simulink model "Pt_All_4WD_TS801"  (Simulink 5.0)
settings: Solver=ode45  StartTime=0  StopTime=25  FixedStep=TSTEP  RelTol=1e-3
PreLoadFcn:
  | cd Extensions/Simulink/pt_all4wd
  | pt_parame_ft4wd
  | cd ../../..
values from neighbouring files (symbols this model uses):
  MENGINE_CARPET = [ ... (first row only)    [mengine_carpet.m]
undefined symbols (not defined in the file or in its folder): AV_ENG_IDLE, DOWNSHIFT_TRANS_TABLE_1, DOWNSHIFT_TRANS_TABLE_2, DOWNSHIFT_TRANS_TABLE_3, DOWNSHIFT_TRANS_TABLE_4, DOWNSHIFT_TRANS_TABLE_5, DOWNSHIFT_TRANS_TABLE_6, IENG, INV_CAP_TC_TABLE, ITC_INPUT_SHAFT, LOCKED_FD_DAMP, LOCKED_FD_K, LOCKED_FD_OPT, LOCKED_RD_DAMP, LOCKED_RD_K, LOCKED_RD_OPT, LOCKED_XC_DAMP, LOCKED_XC_K, LOCKED_XC_OPT, M_DIFF_FD_TABLE, M_DIFF_RD_TABLE, M_DIFF_XC_TABLE, R_EFF_F_FD, R_EFF_F_RD, R_EFF_F_XC, R_EFF_R_FD, R_EFF_R_RD, R_EFF_R_XC, R_EFF_TR_F, R_EFF_TR_F_REVERSE, R_EFF_TR_R, R_EFF_TR_R_REVERSE, R_GEAR_FD, R_GEAR_RD, R_GEAR_TR, R_GEAR_TR_REVERSE, R_GEAR_XC, R_REAR_XC, RM_TC_TABLE, UPSHIFT_TRANS_TABLE_1, UPSHIFT_TRANS_TABLE_2, UPSHIFT_TRANS_TABLE_3, UPSHIFT_TRANS_TABLE_4, UPSHIFT_TRANS_TABLE_5, UPSHIFT_TRANS_TABLE_6
libraries: Solver_SF x1
settings Model: LastModifiedBy=ywata  ExtModeTrigMode=oneshot  ExtModeArmWhenConnect=off  SaveTime=off  SaveOutput=off  LimitDataPoints=off  BooleanDataType=off

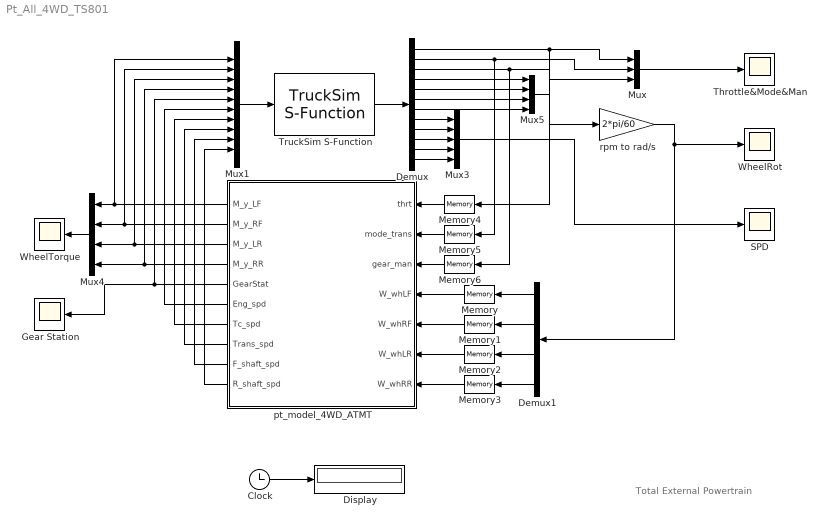
== system Pt_All_4WD_TS801 ==
  note: Total External Powertrain
  Clock : Clock
      settings: Decimation=10
  Demux : Demux  Outputs=12
  Demux1 : Demux  Orientation=left
  Display : Display
  Gear Station : Scope
      settings: YMin=0  YMax=6
  Memory{,1..6} (7 alike) : Memory  Orientation=left
  Mux : Mux  Inputs=3
  Mux1 : Mux  Inputs=10
  Mux3 : Mux  Inputs=5
  Mux4 : Mux  Orientation=left
  Mux5 : Mux
  SPD : Scope
      settings: TimeRange=25  YMin=-50  YMax=100
  Throttle&Mode&Man : Scope
      settings: YMin=0  YMax=7
  TruckSim S-Function : Solver_SF/TruckSim S-Function  Priority=1  AncestorBlock=Solver_SF/CarSim S-Function  VehicleCode=???
      settings: AttributesFormatString=Vehicle Code: %<VehicleCode>
  WheelRot : Scope
      settings: TimeRange=20  YMin=-10  YMax=50
  WheelTorque : Scope
      settings: YMin=0  YMax=2750
  pt_model_4WD_ATMT : Subsystem  Orientation=left
  rpm to rad/s : Gain  Gain=2*pi/60  SaturateOnIntegerOverflow=on
  wires:
  Mux1/1 -> TruckSim S-Function/1
  Mux/1 -> Throttle&Mode&Man/1
  Mux4/1 -> WheelTorque/1
  Demux/1 -> Mux/1, Memory4/1
  Demux/2 -> Mux/2, Memory5/1
  Demux/3 -> Mux/3, Memory6/1
  Demux1/1 -> Memory/1
  Demux1/2 -> Memory1/1
  Demux1/3 -> Memory2/1
  Demux1/4 -> Memory3/1
  Demux/5 -> Mux5/2
  Demux/6 -> Mux5/3
  Demux/4 -> Mux5/1
  Demux/7 -> Mux5/4
  Mux5/1 -> rpm to rad/s/1
  rpm to rad/s/1 -> Demux1/1, WheelRot/1
  Demux/8 -> Mux3/1
  Demux/9 -> Mux3/2
  Demux/10 -> Mux3/3
  Demux/11 -> Mux3/4
  Demux/12 -> Mux3/5
  Mux3/1 -> SPD/1
  pt_model_4WD_ATMT/1(M_y_LF) -> Mux1/1, Mux4/1
  pt_model_4WD_ATMT/2(M_y_RF) -> Mux1/2, Mux4/2
  pt_model_4WD_ATMT/3(M_y_LR) -> Mux4/3, Mux1/3
  pt_model_4WD_ATMT/4(M_y_RR) -> Mux4/4, Mux1/4
  pt_model_4WD_ATMT/5(GearStat) -> Gear Station/1, Mux1/5
  Clock/1 -> Display/1
  TruckSim S-Function/1 -> Demux/1
  Memory/1 -> pt_model_4WD_ATMT/4(W_whLF)
  Memory1/1 -> pt_model_4WD_ATMT/5(W_whRF)
  Memory2/1 -> pt_model_4WD_ATMT/6(W_whLR)
  Memory3/1 -> pt_model_4WD_ATMT/7(W_whRR)
  Memory4/1 -> pt_model_4WD_ATMT/1(thrt)
  Memory5/1 -> pt_model_4WD_ATMT/2(mode_trans)
  Memory6/1 -> pt_model_4WD_ATMT/3(gear_man)
  pt_model_4WD_ATMT/6(Eng_spd) -> Mux1/6
  pt_model_4WD_ATMT/7(Tc_spd) -> Mux1/7
  pt_model_4WD_ATMT/8(Trans_spd) -> Mux1/8
  pt_model_4WD_ATMT/9(F_shaft_spd) -> Mux1/9
  pt_model_4WD_ATMT/10(R_shaft_spd) -> Mux1/10

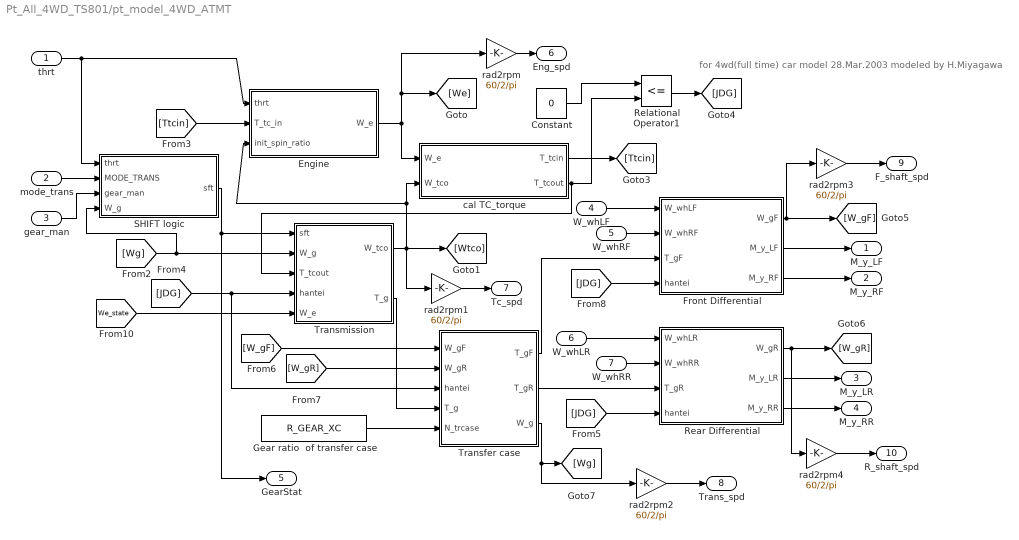
== system Pt_All_4WD_TS801/pt_model_4WD_ATMT ==
  note: for 4wd(full time) car model
      | 28.Mar.2003
      | modeled by H.Miyagawa
  thrt : Inport
  mode_trans : Inport  Port=2
  gear_man : Inport  Port=3
  W_whLF : Inport  Port=4
  W_whRF : Inport  Port=5
  W_whLR : Inport  Port=6
  W_whRR : Inport  Port=7
  Constant : Constant  Value=0
  Engine : Subsystem
  "Front Differential " : Subsystem
  Gear ratio  of transfer case : Constant  Value=R_GEAR_XC
  Rear Differential : Subsystem
  Relational Operator1 : RelationalOperator  Operator=<=  InputSameDT=on
  SHIFT logic : Subsystem
  Transfer case : Subsystem
  Transmission : Subsystem
  cal TC_torque : Subsystem
  rad2rpm{,1..4} (5 alike) : Gain  Gain=60/2/pi  SaturateOnIntegerOverflow=on
  M_y_LF : Outport
  M_y_RF : Outport  Port=2
  M_y_LR : Outport  Port=3
  M_y_RR : Outport  Port=4
  GearStat : Outport  Port=5
  Eng_spd : Outport  Port=6
  Tc_spd : Outport  Port=7
  Trans_spd : Outport  Port=8
  F_shaft_spd : Outport  Port=9
  R_shaft_spd : Outport  Port=10
  wires:
  SHIFT logic/1(sft) -> GearStat/1, Transmission/1(sft)
  [We_state] -> Transmission/5(W_e)
  Gear ratio  of transfer case/1 -> Transfer case/5(N_trcase)
  [W_gR] -> Transfer case/2(W_gR)
  [W_gF] -> Transfer case/1(W_gF)
  Transmission/2(T_g) -> Transfer case/4(T_g)
  [JDG] -> "Front Differential "/4(hantei)
  W_whLF/1 -> "Front Differential "/1(W_whLF)
  W_whRF/1 -> "Front Differential "/2(W_whRF)
  [JDG] -> Transfer case/3(hantei), Transmission/4(hantei)
  Transfer case/1(T_gF) -> "Front Differential "/3(T_gF)
  "Front Differential "/3(M_y_RF) -> M_y_RF/1
  "Front Differential "/2(M_y_LF) -> M_y_LF/1
  cal TC_torque/1(T_tcin) -> [Ttcin]
  cal TC_torque/2(T_tcout) -> Transmission/3(T_tcout), Relational Operator1/2
  [Wg] -> SHIFT logic/4(W_g), Transmission/2(W_g)
  Relational Operator1/1 -> [JDG]
  [Ttcin] -> Engine/2(T_tc_in)
  Transmission/1(W_tco) -> cal TC_torque/2(W_tco), Engine/3(init_spin_ratio), [Wtco], rad2rpm1/1
  Engine/1(W_e) -> cal TC_torque/1(W_e), [We], rad2rpm/1
  mode_trans/1 -> SHIFT logic/2(MODE_TRANS)
  gear_man/1 -> SHIFT logic/3(gear_man)
  thrt/1 -> SHIFT logic/1(thrt), Engine/1(thrt)
  Transfer case/3(W_g) -> [Wg], rad2rpm2/1
  "Front Differential "/1(W_gF) -> [W_gF], rad2rpm3/1
  Transfer case/2(T_gR) -> Rear Differential/3(T_gR)
  Rear Differential/3(M_y_RR) -> M_y_RR/1
  Rear Differential/2(M_y_LR) -> M_y_LR/1
  W_whRR/1 -> Rear Differential/2(W_whRR)
  W_whLR/1 -> Rear Differential/1(W_whLR)
  [JDG] -> Rear Differential/4(hantei)
  Rear Differential/1(W_gR) -> [W_gR], rad2rpm4/1
  rad2rpm/1 -> Eng_spd/1
  rad2rpm1/1 -> Tc_spd/1
  rad2rpm2/1 -> Trans_spd/1
  rad2rpm3/1 -> F_shaft_spd/1
  rad2rpm4/1 -> R_shaft_spd/1
  Constant/1 -> Relational Operator1/1

== system Pt_All_4WD_TS801/pt_model_4WD_ATMT/Engine ==
  thrt : Inport
  T_tc_in : Inport  Port=2
  init_spin_ratio : Inport  Port=3
  Spin inertia of engine crankshaft (kg-m2) : Constant  Value=IENG
  Spin inertia of input shaft of torque converter (kg-m2) : Constant  Value=ITC_INPUT_SHAFT
  cal Engine_torque : Subsystem
  cal We : Subsystem
  W_e : Outport
  wires:
  cal Engine_torque/1(T_e) -> cal We/1(T_e)
  cal We/1(We) -> W_e/1, cal Engine_torque/1(We)
  thrt/1 -> cal Engine_torque/2(thrt)
  init_spin_ratio/1 -> cal We/5(init spin ratio)
  T_tc_in/1 -> cal We/2(T_tc_in)
  Spin inertia of input shaft of torque converter (kg-m2)/1 -> cal We/4(I_tc_in)
  Spin inertia of engine crankshaft (kg-m2)/1 -> cal We/3(I_e)

== system Pt_All_4WD_TS801/pt_model_4WD_ATMT/Front Differential  ==
  W_whLF : Inport
  W_whRF : Inport  Port=2
  T_gF : Inport  Port=3
  hantei : Inport  Port=4
  Differeneial Gear : Subsystem
  Gear ratio of front differential : Constant  Value=R_GEAR_FD
  haibun : Subsystem
  W_gF : Outport
  M_y_LF : Outport  Port=2
  M_y_RF : Outport  Port=3
  wires:
  haibun/2(M_y_RF) -> M_y_RF/1
  haibun/1(M_y_LF) -> M_y_LF/1
  W_whRF/1 -> Differeneial Gear/2(W_whRF), haibun/2(W_whRF)
  W_whLF/1 -> Differeneial Gear/1(W_whLF), haibun/1(W_whLF)
  Gear ratio of front differential/1 -> haibun/5(N_diff_F), Differeneial Gear/3(N_diff_F)
  Differeneial Gear/1(W_g) -> W_gF/1
  T_gF/1 -> haibun/4(T_gF)
  hantei/1 -> haibun/3(hantei)

== system Pt_All_4WD_TS801/pt_model_4WD_ATMT/Rear Differential ==
  W_whLR : Inport
  W_whRR : Inport  Port=2
  T_gR : Inport  Port=3
  hantei : Inport  Port=4
  Differeneial Gear : Subsystem
  Gear ratio of rear differential : Constant  Value=R_GEAR_RD
  haibun : Subsystem
  W_gR : Outport
  M_y_LR : Outport  Port=2
  M_y_RR : Outport  Port=3
  wires:
  hantei/1 -> haibun/3(hantei)
  T_gR/1 -> haibun/4(T_gR)
  Differeneial Gear/1(W_g) -> W_gR/1
  Gear ratio of rear differential/1 -> Differeneial Gear/3(N_diff_R), haibun/5(N_diff_R)
  W_whLR/1 -> haibun/1(W_whLR), Differeneial Gear/1(W_whLR)
  W_whRR/1 -> haibun/2(W_whRR), Differeneial Gear/2(W_whRR)
  haibun/1(M_y_LR) -> M_y_LR/1
  haibun/2(M_y_RR) -> M_y_RR/1

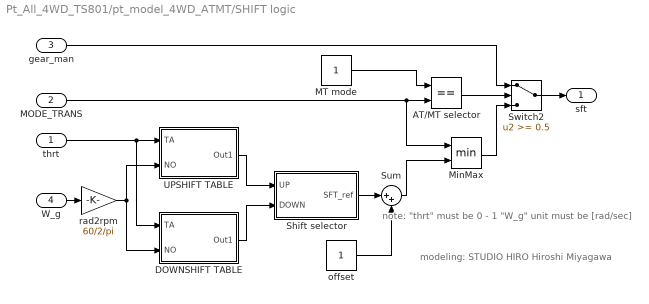
== system Pt_All_4WD_TS801/pt_model_4WD_ATMT/SHIFT logic ==
  note: note:
      | "thrt" must be 0 - 1
      | "W_g" unit must be [rad/sec]
  note: modeling:
      | STUDIO HIRO
      | Hiroshi Miyagawa
  thrt : Inport
  MODE_TRANS : Inport  Port=2
  gear_man : Inport  Port=3
  W_g : Inport  Port=4
  AT/MT selector : RelationalOperator  Operator===  InputSameDT=on
  DOWNSHIFT TABLE : Subsystem
  MT mode : Constant
  MinMax : MinMax  Inputs=2
  Shift selector : Subsystem
  Sum : Sum  Inputs=|++  SaturateOnIntegerOverflow=on  InputSameDT=on
  Switch2 : Switch  Threshold=0.5  SaturateOnIntegerOverflow=on  InputSameDT=on
  UPSHIFT TABLE : Subsystem
  offset : Constant
  rad2rpm : Gain  Gain=60/2/pi  SaturateOnIntegerOverflow=on
  sft : Outport
  wires:
  MinMax/1 -> Switch2/3
  AT/MT selector/1 -> Switch2/2
  gear_man/1 -> Switch2/1
  MODE_TRANS/1 -> MinMax/1, AT/MT selector/2
  MT mode/1 -> AT/MT selector/1
  thrt/1 -> DOWNSHIFT TABLE/1(TA), UPSHIFT TABLE/1(TA)
  Sum/1 -> MinMax/2
  W_g/1 -> rad2rpm/1
  DOWNSHIFT TABLE/1(Out1) -> Shift selector/2(DOWN)
  UPSHIFT TABLE/1(Out1) -> Shift selector/1(UP)
  rad2rpm/1 -> DOWNSHIFT TABLE/2(NO), UPSHIFT TABLE/2(NO)
  Shift selector/1(SFT_ref) -> Sum/1
  offset/1 -> Sum/2
  Switch2/1 -> sft/1

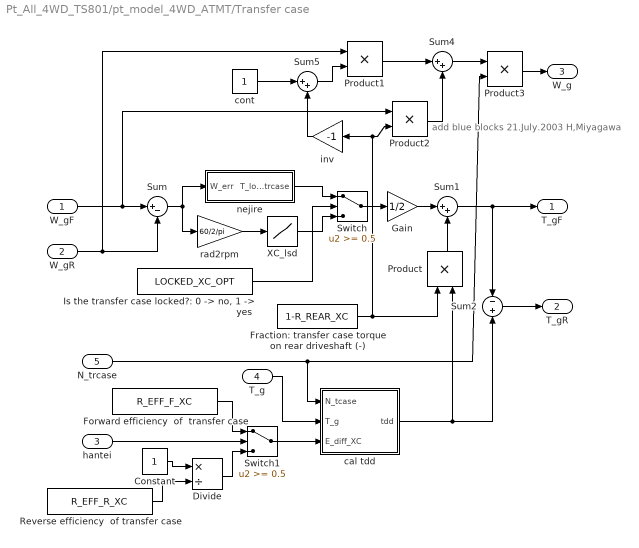
== system Pt_All_4WD_TS801/pt_model_4WD_ATMT/Transfer case ==
  note: add blue blocks
      | 21.July.2003
      | H,Miyagawa
  W_gF : Inport
  W_gR : Inport  Port=2
  hantei : Inport  Port=3
  T_g : Inport  Port=4
  N_trcase : Inport  Port=5
  Constant : Constant
  Divide : Product  Inputs=*/  InputSameDT=on
  Forward efficiency  of  transfer case : Constant  Value=R_EFF_F_XC
  Fraction: transfer case torque on rear driveshaft (-) : Constant  Value=1-R_REAR_XC
  Gain : Gain  Gain=1/2  SaturateOnIntegerOverflow=on
  "Is the transfer case locked?: 0 -> no, 1 -> yes" : Constant  Value=LOCKED_XC_OPT
  Product : Product  Orientation=up  SaturateOnIntegerOverflow=on  InputSameDT=on
  Product1 : Product  SaturateOnIntegerOverflow=on  InputSameDT=on
  Product2 : Product  SaturateOnIntegerOverflow=on  InputSameDT=on
  Product3 : Product  SaturateOnIntegerOverflow=on  InputSameDT=on
  Reverse efficiency  of transfer case : Constant  Value=R_EFF_R_XC
  Sum : Sum  Inputs=|+-  SaturateOnIntegerOverflow=on  InputSameDT=on
  Sum1 : Sum  Inputs=|++  SaturateOnIntegerOverflow=on  InputSameDT=on
  Sum2 : Sum  Inputs=-|+  SaturateOnIntegerOverflow=on  InputSameDT=on
  Sum4 : Sum  Inputs=|++  SaturateOnIntegerOverflow=on  InputSameDT=on
  Sum5 : Sum  Inputs=|++  SaturateOnIntegerOverflow=on  InputSameDT=on
  Switch : Switch  Threshold=0.5  SaturateOnIntegerOverflow=on  InputSameDT=on
  Switch1 : Switch  Threshold=0.5  SaturateOnIntegerOverflow=on  InputSameDT=on
  XC_lsd : Lookup  InputValues=M_DIFF_XC_TABLE(:,1)  OutputValues=M_DIFF_XC_TABLE(:,2)  SaturateOnIntegerOverflow=on
  cal tdd : Subsystem
  cont : Constant
  inv : Gain  Orientation=left  Gain=-1  SaturateOnIntegerOverflow=on
  nejire : Subsystem
  rad2rpm : Gain  Gain=60/2/pi  SaturateOnIntegerOverflow=on
  T_gF : Outport
  T_gR : Outport  Port=2
  W_g : Outport  Port=3
  wires:
  Sum1/1 -> Sum2/1, T_gF/1
  Sum2/1 -> T_gR/1
  cal tdd/1(tdd) -> Product/2, Sum2/2
  Switch1/1 -> cal tdd/3(E_diff_XC)
  Forward efficiency  of  transfer case/1 -> Switch1/1
  hantei/1 -> Switch1/2
  T_g/1 -> cal tdd/2(T_g)
  Product/1 -> Sum1/2
  Gain/1 -> Sum1/1
  Switch/1 -> Gain/1
  XC_lsd/1 -> Switch/3
  "Is the transfer case locked?: 0 -> no, 1 -> yes"/1 -> Switch/2
  Sum/1 -> rad2rpm/1, nejire/1(W_err)
  rad2rpm/1 -> XC_lsd/1
  nejire/1(T_lock_trcase) -> Switch/1
  Fraction: transfer case torque on rear driveshaft (-)/1 -> Product/1, Product2/2, inv/1
  Product2/1 -> Sum4/2
  Product1/1 -> Sum4/1
  Sum4/1 -> Product3/1
  Product3/1 -> W_g/1
  N_trcase/1 -> cal tdd/1(N_tcase), Product3/2
  Sum5/1 -> Product1/2
  cont/1 -> Sum5/1
  inv/1 -> Sum5/2
  W_gF/1 -> Sum/1, Product2/1
  W_gR/1 -> Sum/2, Product1/1
  Constant/1 -> Divide/1
  Reverse efficiency  of transfer case/1 -> Divide/2
  Divide/1 -> Switch1/3

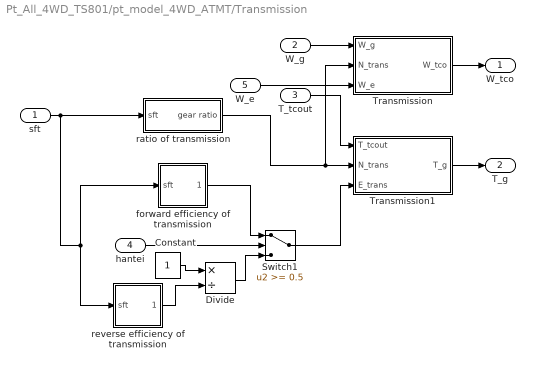
== system Pt_All_4WD_TS801/pt_model_4WD_ATMT/Transmission ==
  sft : Inport
  W_g : Inport  Port=2
  T_tcout : Inport  Port=3
  hantei : Inport  Port=4
  W_e : Inport  Port=5
  Constant : Constant
  Divide : Product  Inputs=*/  InputSameDT=on
  Switch1 : Switch  Threshold=0.5  SaturateOnIntegerOverflow=on  InputSameDT=on
  Transmission : Subsystem
  Transmission1 : Subsystem
  forward efficiency of transmission : Subsystem  mask(forward efficiency of transmission){data=R_EFF_TR_F, data_rev=R_EFF_TR_F_REVERSE}
      mask prompts: data "gear"; data_rev "Reverse-gear"
  ratio of transmission : Subsystem  mask(forward efficiency of transmission){data=R_GEAR_TR, data_rev=R_GEAR_TR_REVERSE}
      mask prompts: data "gear ratio"; data_rev "Reverse-gear ratio"
      mask help:
      | input:
      |  sft is must be 0 - 7
      | output:
      |  transmission gear ratio
      |  when Nutral(0), it is zero
      | 1st parameta:
      |  must be vector
      | 2nd parameter:
      |  should be negative
  reverse efficiency of transmission : Subsystem  mask(reverse efficiency of transmission){data=R_EFF_TR_R, data_rev=R_EFF_TR_R_REVERSE}
      mask prompts: data "gear"; data_rev "Reverse-gear"
  W_tco : Outport
  T_g : Outport  Port=2
  wires:
  W_e/1 -> Transmission/3(W_e)
  forward efficiency of transmission/1(Out1) -> Switch1/1
  hantei/1 -> Switch1/2
  ratio of transmission/1(gear ratio) -> Transmission1/2(N_trans), Transmission/2(N_trans)
  W_g/1 -> Transmission/1(W_g)
  Transmission1/1(T_g) -> T_g/1
  T_tcout/1 -> Transmission1/1(T_tcout)
  Switch1/1 -> Transmission1/3(E_trans)
  sft/1 -> ratio of transmission/1(sft), reverse efficiency of transmission/1(sft), forward efficiency of transmission/1(sft)
  Transmission/1(W_tco) -> W_tco/1
  Constant/1 -> Divide/1
  reverse efficiency of transmission/1(Out1) -> Divide/2
  Divide/1 -> Switch1/3

== system Pt_All_4WD_TS801/pt_model_4WD_ATMT/cal TC_torque ==
  note: Torque Convertor input & output torque calculation
  W_e : Inport
  W_tco : Inport  Port=2
  Math Function : Math  Operator=square
  Product : Product  SaturateOnIntegerOverflow=on  InputSameDT=on
  Product1 : Product  SaturateOnIntegerOverflow=on  InputSameDT=on
  Product2 : Product  SaturateOnIntegerOverflow=on  InputSameDT=on
  Sign : Signum
  cal speed_ratio : Subsystem
  f_tki : Lookup  InputValues=INV_CAP_TC_TABLE(:,1)  OutputValues=INV_CAP_TC_TABLE(:,2)  SaturateOnIntegerOverflow=on
  f_tr : Lookup  InputValues=RM_TC_TABLE(:,1)  OutputValues=RM_TC_TABLE(:,2)  SaturateOnIntegerOverflow=on
  rad2rpm : Gain  Gain=60/2/pi  SaturateOnIntegerOverflow=on
  T_tcin : Outport
  T_tcout : Outport  Port=2
  wires:
  Product/1 -> Math Function/1
  f_tki/1 -> Product/1, Sign/1
  Math Function/1 -> Product1/2
  Sign/1 -> Product1/1
  W_e/1 -> cal speed_ratio/2(W_e), rad2rpm/1
  cal speed_ratio/1(S_tc) -> f_tki/1, f_tr/1
  f_tr/1 -> Product2/2
  Product1/1 -> Product2/1, T_tcin/1
  W_tco/1 -> cal speed_ratio/1(W_tco)
  Product2/1 -> T_tcout/1
  rad2rpm/1 -> Product/2

== system Pt_All_4WD_TS801/pt_model_4WD_ATMT/Engine/cal Engine_torque ==
  We : Inport
  thrt : Inport  Port=2
  f_et : Lookup2D  RowIndex=MENGINE_CARPET(2:18,1)  ColumnIndex=MENGINE_CARPET(1,2:12)  OutputValues=MENGINE_CARPET(2:18,2:12)  SaturateOnIntegerOverflow=on  InputSameDT=on
  rad2rpm : Gain  Gain=60/2/pi  SaturateOnIntegerOverflow=on
  T_e : Outport
  wires:
  rad2rpm/1 -> f_et/1
  We/1 -> rad2rpm/1
  f_et/1 -> T_e/1
  thrt/1 -> f_et/2

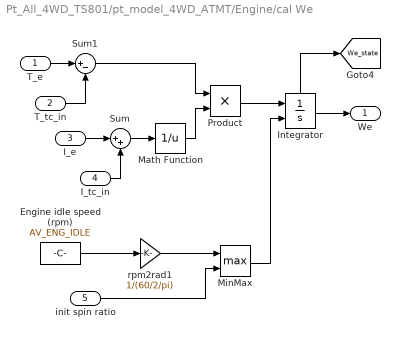
== system Pt_All_4WD_TS801/pt_model_4WD_ATMT/Engine/cal We ==
  T_e : Inport
  T_tc_in : Inport  Port=2
  I_e : Inport  Port=3
  I_tc_in : Inport  Port=4
  init spin ratio : Inport  Port=5
  Engine idle speed (rpm) : Constant  Value=AV_ENG_IDLE
  Integrator : Integrator  InitialConditionSource=external  InitialCondition=AV_ENG_IDLE*2*pi/60  ShowStatePort=on
  Math Function : Math  Operator=reciprocal
  MinMax : MinMax  Function=max  Inputs=2
  Product : Product  SaturateOnIntegerOverflow=on  InputSameDT=on
  Sum : Sum  Inputs=|++  SaturateOnIntegerOverflow=on  InputSameDT=on
  Sum1 : Sum  Inputs=|+-  SaturateOnIntegerOverflow=on  InputSameDT=on
  rpm2rad1 : Gain  Gain=1/(60/2/pi)  SaturateOnIntegerOverflow=on
  We : Outport
  tag scope: We_state=global
  wires:
  Integrator/State -> [We_state]
  MinMax/1 -> Integrator/2
  rpm2rad1/1 -> MinMax/1
  Engine idle speed (rpm)/1 -> rpm2rad1/1
  init spin ratio/1 -> MinMax/2
  Integrator/1 -> We/1
  Product/1 -> Integrator/1
  I_tc_in/1 -> Sum/2
  I_e/1 -> Sum/1
  T_tc_in/1 -> Sum1/2
  Sum/1 -> Math Function/1
  T_e/1 -> Sum1/1
  Sum1/1 -> Product/1
  Math Function/1 -> Product/2

== system Pt_All_4WD_TS801/pt_model_4WD_ATMT/Front Differential /Differeneial Gear ==
  W_whLF : Inport
  W_whRF : Inport  Port=2
  N_diff_F : Inport  Port=3
  Gain1 : Gain  Gain=1/2  SaturateOnIntegerOverflow=on
  Product : Product  SaturateOnIntegerOverflow=on  InputSameDT=on
  Sum : Sum  Inputs=|++  SaturateOnIntegerOverflow=on  InputSameDT=on
  W_g : Outport
  wires:
  Product/1 -> W_g/1
  Gain1/1 -> Product/1
  W_whRF/1 -> Sum/2
  W_whLF/1 -> Sum/1
  N_diff_F/1 -> Product/2
  Sum/1 -> Gain1/1

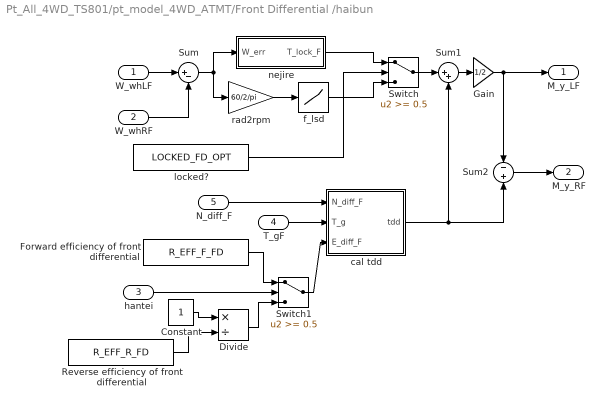
== system Pt_All_4WD_TS801/pt_model_4WD_ATMT/Front Differential /haibun ==
  W_whLF : Inport
  W_whRF : Inport  Port=2
  hantei : Inport  Port=3
  T_gF : Inport  Port=4
  N_diff_F : Inport  Port=5
  Constant : Constant
  Divide : Product  Inputs=*/  InputSameDT=on
  Forward efficiency of front differential : Constant  Value=R_EFF_F_FD
  Gain : Gain  Gain=1/2  SaturateOnIntegerOverflow=on
  Reverse efficiency of front differential : Constant  Value=R_EFF_R_FD
  Sum : Sum  Inputs=|+-  SaturateOnIntegerOverflow=on  InputSameDT=on
  Sum1 : Sum  Inputs=|++  SaturateOnIntegerOverflow=on  InputSameDT=on
  Sum2 : Sum  Inputs=-|+  SaturateOnIntegerOverflow=on  InputSameDT=on
  Switch : Switch  Threshold=0.5  SaturateOnIntegerOverflow=on  InputSameDT=on
  Switch1 : Switch  Threshold=0.5  SaturateOnIntegerOverflow=on  InputSameDT=on
  cal tdd : Subsystem
  f_lsd : Lookup  InputValues=M_DIFF_FD_TABLE(:,1)  OutputValues=M_DIFF_FD_TABLE(:,2)  SaturateOnIntegerOverflow=on
  locked? : Constant  Value=LOCKED_FD_OPT
  nejire : Subsystem
  rad2rpm : Gain  Gain=60/2/pi  SaturateOnIntegerOverflow=on
  M_y_LF : Outport
  M_y_RF : Outport  Port=2
  wires:
  T_gF/1 -> cal tdd/2(T_g)
  hantei/1 -> Switch1/2
  Forward efficiency of front differential/1 -> Switch1/1
  Switch1/1 -> cal tdd/3(E_diff_F)
  W_whLF/1 -> Sum/1
  W_whRF/1 -> Sum/2
  cal tdd/1(tdd) -> Sum1/2, Sum2/2
  Sum2/1 -> M_y_RF/1
  N_diff_F/1 -> cal tdd/1(N_diff_F)
  nejire/1(T_lock_F) -> Switch/1
  Switch/1 -> Sum1/1
  rad2rpm/1 -> f_lsd/1
  Sum1/1 -> Gain/1
  Gain/1 -> M_y_LF/1, Sum2/1
  Sum/1 -> nejire/1(W_err), rad2rpm/1
  locked?/1 -> Switch/2
  f_lsd/1 -> Switch/3
  Constant/1 -> Divide/1
  Reverse efficiency of front differential/1 -> Divide/2
  Divide/1 -> Switch1/3

== system Pt_All_4WD_TS801/pt_model_4WD_ATMT/Rear Differential/Differeneial Gear ==
  W_whLR : Inport
  W_whRR : Inport  Port=2
  N_diff_R : Inport  Port=3
  Gain1 : Gain  Gain=1/2  SaturateOnIntegerOverflow=on
  Product : Product  SaturateOnIntegerOverflow=on  InputSameDT=on
  Sum : Sum  Inputs=|++  SaturateOnIntegerOverflow=on  InputSameDT=on
  W_g : Outport
  wires:
  Sum/1 -> Gain1/1
  N_diff_R/1 -> Product/2
  W_whLR/1 -> Sum/1
  W_whRR/1 -> Sum/2
  Gain1/1 -> Product/1
  Product/1 -> W_g/1

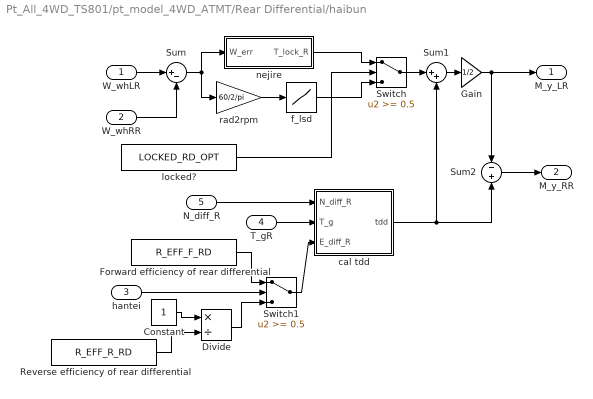
== system Pt_All_4WD_TS801/pt_model_4WD_ATMT/Rear Differential/haibun ==
  W_whLR : Inport
  W_whRR : Inport  Port=2
  hantei : Inport  Port=3
  T_gR : Inport  Port=4
  N_diff_R : Inport  Port=5
  Constant : Constant
  Divide : Product  Inputs=*/  InputSameDT=on
  Forward efficiency of rear differential : Constant  Value=R_EFF_F_RD
  Gain : Gain  Gain=1/2  SaturateOnIntegerOverflow=on
  Reverse efficiency of rear differential : Constant  Value=R_EFF_R_RD
  Sum : Sum  Inputs=|+-  SaturateOnIntegerOverflow=on  InputSameDT=on
  Sum1 : Sum  Inputs=|++  SaturateOnIntegerOverflow=on  InputSameDT=on
  Sum2 : Sum  Inputs=-|+  SaturateOnIntegerOverflow=on  InputSameDT=on
  Switch : Switch  Threshold=0.5  SaturateOnIntegerOverflow=on  InputSameDT=on
  Switch1 : Switch  Threshold=0.5  SaturateOnIntegerOverflow=on  InputSameDT=on
  cal tdd : Subsystem
  f_lsd : Lookup  InputValues=M_DIFF_RD_TABLE(:,1)  OutputValues=M_DIFF_RD_TABLE(:,2)  SaturateOnIntegerOverflow=on
  locked? : Constant  Value=LOCKED_RD_OPT
  nejire : Subsystem
  rad2rpm : Gain  Gain=60/2/pi  SaturateOnIntegerOverflow=on
  M_y_LR : Outport
  M_y_RR : Outport  Port=2
  wires:
  f_lsd/1 -> Switch/3
  locked?/1 -> Switch/2
  Sum/1 -> rad2rpm/1, nejire/1(W_err)
  Gain/1 -> Sum2/1, M_y_LR/1
  Sum1/1 -> Gain/1
  rad2rpm/1 -> f_lsd/1
  Switch/1 -> Sum1/1
  nejire/1(T_lock_R) -> Switch/1
  N_diff_R/1 -> cal tdd/1(N_diff_R)
  Sum2/1 -> M_y_RR/1
  cal tdd/1(tdd) -> Sum2/2, Sum1/2
  W_whRR/1 -> Sum/2
  W_whLR/1 -> Sum/1
  Switch1/1 -> cal tdd/3(E_diff_R)
  Forward efficiency of rear differential/1 -> Switch1/1
  hantei/1 -> Switch1/2
  T_gR/1 -> cal tdd/2(T_g)
  Constant/1 -> Divide/1
  Reverse efficiency of rear differential/1 -> Divide/2
  Divide/1 -> Switch1/3

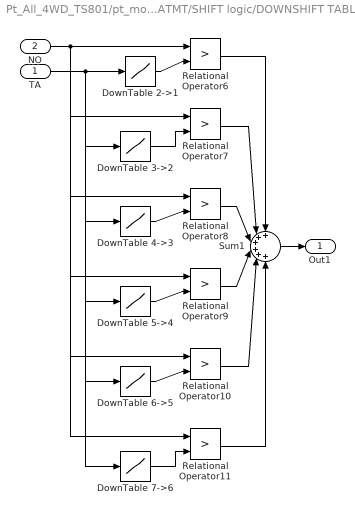
== system Pt_All_4WD_TS801/pt_model_4WD_ATMT/SHIFT logic/DOWNSHIFT TABLE ==
  TA : Inport
  NO : Inport  Port=2
  DownTable 2->1 : Lookup  InputValues=DOWNSHIFT_TRANS_TABLE_1(:,1)  OutputValues=DOWNSHIFT_TRANS_TABLE_1(:,2)  SaturateOnIntegerOverflow=on
  DownTable 3->2 : Lookup  InputValues=DOWNSHIFT_TRANS_TABLE_2(:,1)  OutputValues=DOWNSHIFT_TRANS_TABLE_2(:,2)  SaturateOnIntegerOverflow=on
  DownTable 4->3 : Lookup  InputValues=DOWNSHIFT_TRANS_TABLE_3(:,1)  OutputValues=DOWNSHIFT_TRANS_TABLE_3(:,2)  SaturateOnIntegerOverflow=on
  DownTable 5->4 : Lookup  InputValues=DOWNSHIFT_TRANS_TABLE_4(:,1)  OutputValues=DOWNSHIFT_TRANS_TABLE_4(:,2)  SaturateOnIntegerOverflow=on
  DownTable 6->5 : Lookup  InputValues=DOWNSHIFT_TRANS_TABLE_5(:,1)  OutputValues=DOWNSHIFT_TRANS_TABLE_5(:,2)  SaturateOnIntegerOverflow=on
  DownTable 7->6 : Lookup  InputValues=DOWNSHIFT_TRANS_TABLE_6(:,1)  OutputValues=DOWNSHIFT_TRANS_TABLE_6(:,2)  SaturateOnIntegerOverflow=on
  Relational Operator{6..11} (6 alike) : RelationalOperator  Operator=>  InputSameDT=on
  Sum1 : Sum  Inputs=6  SaturateOnIntegerOverflow=on  InputSameDT=on
  Out1 : Outport
  wires:
  Sum1/1 -> Out1/1
  NO/1 -> Relational Operator11/1, Relational Operator10/1, Relational Operator9/1, Relational Operator8/1, Relational Operator7/1, Relational Operator6/1
  TA/1 -> DownTable 7->6/1, DownTable 6->5/1, DownTable 5->4/1, DownTable 4->3/1, DownTable 3->2/1, DownTable 2->1/1
  DownTable 7->6/1 -> Relational Operator11/2
  DownTable 6->5/1 -> Relational Operator10/2
  DownTable 5->4/1 -> Relational Operator9/2
  DownTable 3->2/1 -> Relational Operator7/2
  DownTable 2->1/1 -> Relational Operator6/2
  Relational Operator11/1 -> Sum1/6
  Relational Operator10/1 -> Sum1/5
  Relational Operator9/1 -> Sum1/4
  Relational Operator8/1 -> Sum1/3
  Relational Operator7/1 -> Sum1/2
  Relational Operator6/1 -> Sum1/1
  DownTable 4->3/1 -> Relational Operator8/2

== system Pt_All_4WD_TS801/pt_model_4WD_ATMT/SHIFT logic/Shift selector ==
  UP : Inport
  DOWN : Inport  Port=2
  Logical Operator2 : Logic  Operator=OR
  Memory : Memory  Orientation=left
  Relational Operator2 : RelationalOperator  Operator=>  InputSameDT=on
  Relational Operator3 : RelationalOperator  Operator=>  InputSameDT=on
  Switch : Switch  Threshold=0.5  SaturateOnIntegerOverflow=on  InputSameDT=on
  Switch1 : Switch  Threshold=0.5  SaturateOnIntegerOverflow=on  InputSameDT=on
  SFT_ref : Outport
  wires:
  DOWN/1 -> Switch1/3, Relational Operator3/2
  UP/1 -> Switch1/1, Relational Operator2/1
  Relational Operator3/1 -> Logical Operator2/2
  Relational Operator2/1 -> Logical Operator2/1, Switch1/2
  Logical Operator2/1 -> Switch/2
  [SFT] -> Relational Operator3/1, Relational Operator2/2
  Memory/1 -> [SFT], Switch/3
  Switch1/1 -> Switch/1
  Switch/1 -> SFT_ref/1, Memory/1

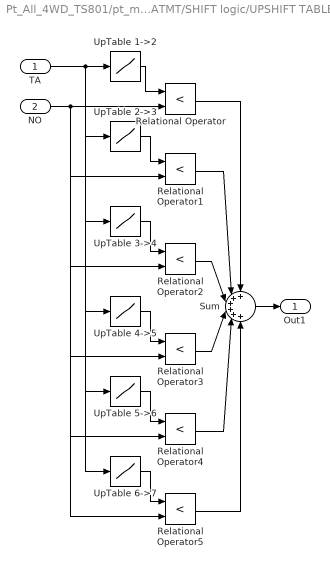
== system Pt_All_4WD_TS801/pt_model_4WD_ATMT/SHIFT logic/UPSHIFT TABLE ==
  TA : Inport
  NO : Inport  Port=2
  Relational Operator{,1..5} (6 alike) : RelationalOperator  Operator=<  InputSameDT=on
  Sum : Sum  Inputs=6  SaturateOnIntegerOverflow=on  InputSameDT=on
  UpTable 1->2 : Lookup  InputValues=UPSHIFT_TRANS_TABLE_1(:,1)  OutputValues=UPSHIFT_TRANS_TABLE_1(:,2)  SaturateOnIntegerOverflow=on
  UpTable 2->3 : Lookup  InputValues=UPSHIFT_TRANS_TABLE_2(:,1)  OutputValues=UPSHIFT_TRANS_TABLE_2(:,2)  SaturateOnIntegerOverflow=on
  UpTable 3->4 : Lookup  InputValues=UPSHIFT_TRANS_TABLE_3(:,1)  OutputValues=UPSHIFT_TRANS_TABLE_3(:,2)  SaturateOnIntegerOverflow=on
  UpTable 4->5 : Lookup  InputValues=UPSHIFT_TRANS_TABLE_4(:,1)  OutputValues=UPSHIFT_TRANS_TABLE_4(:,2)  SaturateOnIntegerOverflow=on
  UpTable 5->6 : Lookup  InputValues=UPSHIFT_TRANS_TABLE_5(:,1)  OutputValues=UPSHIFT_TRANS_TABLE_5(:,2)  SaturateOnIntegerOverflow=on
  UpTable 6->7 : Lookup  InputValues=UPSHIFT_TRANS_TABLE_6(:,1)  OutputValues=UPSHIFT_TRANS_TABLE_6(:,2)  SaturateOnIntegerOverflow=on
  Out1 : Outport
  wires:
  Sum/1 -> Out1/1
  NO/1 -> Relational Operator5/2, Relational Operator4/2, Relational Operator3/2, Relational Operator2/2, Relational Operator1/2, Relational Operator/2
  TA/1 -> UpTable 6->7/1, UpTable 5->6/1, UpTable 4->5/1, UpTable 3->4/1, UpTable 2->3/1, UpTable 1->2/1
  Relational Operator5/1 -> Sum/6
  Relational Operator4/1 -> Sum/5
  Relational Operator3/1 -> Sum/4
  Relational Operator2/1 -> Sum/3
  Relational Operator1/1 -> Sum/2
  Relational Operator/1 -> Sum/1
  UpTable 6->7/1 -> Relational Operator5/1
  UpTable 5->6/1 -> Relational Operator4/1
  UpTable 4->5/1 -> Relational Operator3/1
  UpTable 3->4/1 -> Relational Operator2/1
  UpTable 2->3/1 -> Relational Operator1/1
  UpTable 1->2/1 -> Relational Operator/1

== system Pt_All_4WD_TS801/pt_model_4WD_ATMT/Transfer case/cal tdd ==
  N_tcase : Inport
  T_g : Inport  Port=2
  E_diff_XC : Inport  Port=3
  Gain : Gain  SaturateOnIntegerOverflow=on
  Product : Product  Inputs=3  SaturateOnIntegerOverflow=on  InputSameDT=on
  tdd : Outport
  wires:
  T_g/1 -> Product/1
  N_tcase/1 -> Product/2
  E_diff_XC/1 -> Product/3
  Product/1 -> Gain/1
  Gain/1 -> tdd/1

== system Pt_All_4WD_TS801/pt_model_4WD_ATMT/Transfer case/nejire ==
  W_err : Inport
  Gain : Gain  Gain=-1  SaturateOnIntegerOverflow=on
  Integrator1 : Integrator
  Product : Product  SaturateOnIntegerOverflow=on  InputSameDT=on
  Product1 : Product  SaturateOnIntegerOverflow=on  InputSameDT=on
  Sum1 : Sum  Inputs=|++  SaturateOnIntegerOverflow=on  InputSameDT=on
  Torsional damping constant for locking the transfer case (N-m-s/deg) : Constant  Value=LOCKED_XC_DAMP
  Torsional spring constant for locking the transfer case (N-m/deg) : Constant  Value=LOCKED_XC_K
  rad2deg : Gain  Gain=360/2/pi  SaturateOnIntegerOverflow=on
  T_lock_trcase : Outport
  wires:
  Torsional spring constant for locking the transfer case (N-m/deg)/1 -> Product1/2
  Integrator1/1 -> Product1/1
  Torsional damping constant for locking the transfer case (N-m-s/deg)/1 -> Product/2
  Product/1 -> Sum1/1
  Product1/1 -> Sum1/2
  Sum1/1 -> Gain/1
  Gain/1 -> T_lock_trcase/1
  W_err/1 -> rad2deg/1
  rad2deg/1 -> Product/1, Integrator1/1

== system Pt_All_4WD_TS801/pt_model_4WD_ATMT/Transmission/Transmission ==
  W_g : Inport
  N_trans : Inport  Port=2
  W_e : Inport  Port=3
  Constant : Constant  Value=0
  Constant1 : Constant  Value=0
  MinMax : MinMax  Function=max  Inputs=2
  Product : Product  SaturateOnIntegerOverflow=on  InputSameDT=on
  Relational Operator : RelationalOperator  Operator===  InputSameDT=on
  Switch : Switch  Threshold=0.5  SaturateOnIntegerOverflow=on  InputSameDT=on
  W_tco : Outport
  wires:
  MinMax/1 -> Switch/3
  Product/1 -> MinMax/1
  Constant1/1 -> MinMax/2
  Switch/1 -> W_tco/1
  N_trans/1 -> Relational Operator/2, Product/1
  Constant/1 -> Relational Operator/1
  W_e/1 -> Switch/1
  Relational Operator/1 -> Switch/2
  W_g/1 -> Product/2

== system Pt_All_4WD_TS801/pt_model_4WD_ATMT/Transmission/Transmission1 ==
  T_tcout : Inport
  N_trans : Inport  Port=2
  E_trans : Inport  Port=3
  Product : Product  Inputs=3  SaturateOnIntegerOverflow=on  InputSameDT=on
  T_g : Outport
  wires:
  N_trans/1 -> Product/2
  T_tcout/1 -> Product/1
  E_trans/1 -> Product/3
  Product/1 -> T_g/1

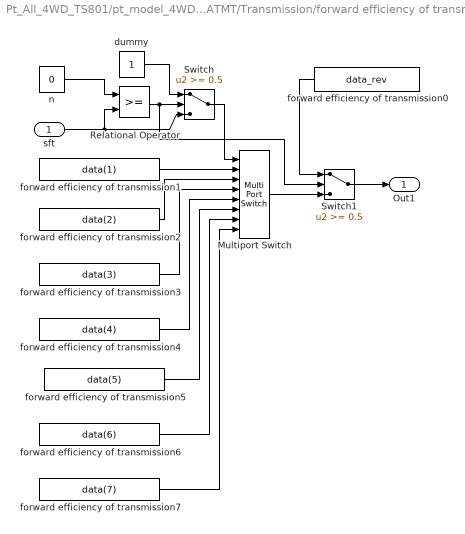
== system Pt_All_4WD_TS801/pt_model_4WD_ATMT/Transmission/forward efficiency of transmission ==
  sft : Inport
  Multiport Switch : MultiPortSwitch  Inputs=7  SaturateOnIntegerOverflow=on  InputSameDT=on
  Relational Operator : RelationalOperator  InputSameDT=on
  Switch : Switch  Threshold=0.5  SaturateOnIntegerOverflow=on  InputSameDT=on
  Switch1 : Switch  Threshold=0.5  SaturateOnIntegerOverflow=on  InputSameDT=on
  dummy : Constant
  forward efficiency of transmission0 : Constant  Orientation=left  Value=data_rev
  forward efficiency of transmission1 : Constant  Value=data(1)
  forward efficiency of transmission2 : Constant  Value=data(2)
  forward efficiency of transmission3 : Constant  Value=data(3)
  forward efficiency of transmission4 : Constant  Value=data(4)
  forward efficiency of transmission5 : Constant  Value=data(5)
  forward efficiency of transmission6 : Constant  Value=data(6)
  forward efficiency of transmission7 : Constant  Value=data(7)
  n : Constant  Value=0
  Out1 : Outport
  wires:
  dummy/1 -> Switch/1
  forward efficiency of transmission0/1 -> Switch1/1
  Relational Operator/1 -> Switch1/2, Switch/2
  n/1 -> Relational Operator/1
  sft/1 -> Switch/3, Relational Operator/2
  Multiport Switch/1 -> Switch1/3
  Switch1/1 -> Out1/1
  forward efficiency of transmission7/1 -> Multiport Switch/8
  forward efficiency of transmission6/1 -> Multiport Switch/7
  forward efficiency of transmission5/1 -> Multiport Switch/6
  forward efficiency of transmission4/1 -> Multiport Switch/5
  forward efficiency of transmission3/1 -> Multiport Switch/4
  forward efficiency of transmission2/1 -> Multiport Switch/3
  Switch/1 -> Multiport Switch/1
  forward efficiency of transmission1/1 -> Multiport Switch/2

== system Pt_All_4WD_TS801/pt_model_4WD_ATMT/Transmission/ratio of transmission ==
  sft : Inport
  1st-gear ratio of transmission : Constant  Value=data(1)
  2nd-gear ratio of transmission2 : Constant  Value=data(2)
  3rd-gear ratio of transmission3 : Constant  Value=data(3)
  4th-gear ratio of transmission4 : Constant  Value=data(4)
  5th-gear ratio of transmission5 : Constant  Value=data(5)
  6th-gear ratio of transmission6 : Constant  Value=data(6)
  7th-gear ratio of transmission7 : Constant  Value=data(7)
  Multiport Switch : MultiPortSwitch  Inputs=9  SaturateOnIntegerOverflow=on  InputSameDT=on
  N : Constant  Value=0
  Reverse-gear ratio of transmission1 : Constant  Value=data_rev
  Sum : Sum  Inputs=2  SaturateOnIntegerOverflow=on  InputSameDT=on
  off set : Constant  Value=2
  gear ratio : Outport
  wires:
  N/1 -> Multiport Switch/3
  Sum/1 -> Multiport Switch/1
  Reverse-gear ratio of transmission1/1 -> Multiport Switch/2
  7th-gear ratio of transmission7/1 -> Multiport Switch/10
  6th-gear ratio of transmission6/1 -> Multiport Switch/9
  5th-gear ratio of transmission5/1 -> Multiport Switch/8
  4th-gear ratio of transmission4/1 -> Multiport Switch/7
  3rd-gear ratio of transmission3/1 -> Multiport Switch/6
  2nd-gear ratio of transmission2/1 -> Multiport Switch/5
  1st-gear ratio of transmission/1 -> Multiport Switch/4
  Multiport Switch/1 -> gear ratio/1
  off set/1 -> Sum/1
  sft/1 -> Sum/2

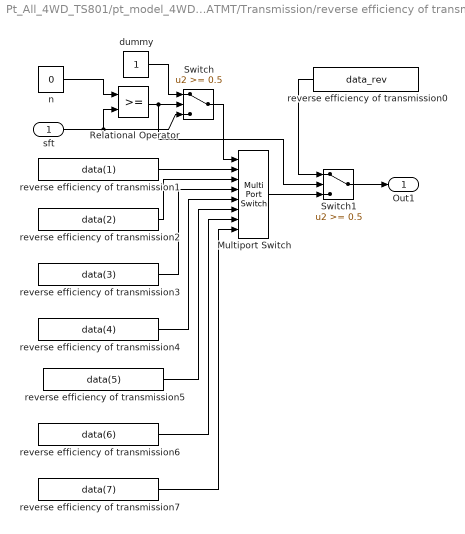
== system Pt_All_4WD_TS801/pt_model_4WD_ATMT/Transmission/reverse efficiency of transmission ==
  sft : Inport
  Multiport Switch : MultiPortSwitch  Inputs=7  SaturateOnIntegerOverflow=on  InputSameDT=on
  Relational Operator : RelationalOperator  InputSameDT=on
  Switch : Switch  Threshold=0.5  SaturateOnIntegerOverflow=on  InputSameDT=on
  Switch1 : Switch  Threshold=0.5  SaturateOnIntegerOverflow=on  InputSameDT=on
  dummy : Constant
  n : Constant  Value=0
  reverse efficiency of transmission0 : Constant  Orientation=left  Value=data_rev
  reverse efficiency of transmission1 : Constant  Value=data(1)
  reverse efficiency of transmission2 : Constant  Value=data(2)
  reverse efficiency of transmission3 : Constant  Value=data(3)
  reverse efficiency of transmission4 : Constant  Value=data(4)
  reverse efficiency of transmission5 : Constant  Value=data(5)
  reverse efficiency of transmission6 : Constant  Value=data(6)
  reverse efficiency of transmission7 : Constant  Value=data(7)
  Out1 : Outport
  wires:
  dummy/1 -> Switch/1
  reverse efficiency of transmission0/1 -> Switch1/1
  reverse efficiency of transmission1/1 -> Multiport Switch/2
  Switch/1 -> Multiport Switch/1
  reverse efficiency of transmission2/1 -> Multiport Switch/3
  reverse efficiency of transmission3/1 -> Multiport Switch/4
  reverse efficiency of transmission4/1 -> Multiport Switch/5
  reverse efficiency of transmission5/1 -> Multiport Switch/6
  reverse efficiency of transmission6/1 -> Multiport Switch/7
  reverse efficiency of transmission7/1 -> Multiport Switch/8
  Switch1/1 -> Out1/1
  Multiport Switch/1 -> Switch1/3
  sft/1 -> Relational Operator/2, Switch/3
  n/1 -> Relational Operator/1
  Relational Operator/1 -> Switch/2, Switch1/2

== system Pt_All_4WD_TS801/pt_model_4WD_ATMT/cal TC_torque/cal speed_ratio ==
  W_tco : Inport
  W_e : Inport  Port=2
  Constant : Constant
  Math Function : Math  Operator=reciprocal
  Product : Product  SaturateOnIntegerOverflow=on  InputSameDT=on
  Switch : Switch  Threshold=1  SaturateOnIntegerOverflow=on  InputSameDT=on
  S_tc : Outport
  wires:
  Math Function/1 -> Product/2
  W_tco/1 -> Product/1
  Product/1 -> S_tc/1
  Switch/1 -> Math Function/1
  W_e/1 -> Switch/1, Switch/2
  Constant/1 -> Switch/3

== system Pt_All_4WD_TS801/pt_model_4WD_ATMT/Front Differential /haibun/cal tdd ==
  N_diff_F : Inport
  T_g : Inport  Port=2
  E_diff_F : Inport  Port=3
  Gain : Gain  SaturateOnIntegerOverflow=on
  Product : Product  Inputs=3  SaturateOnIntegerOverflow=on  InputSameDT=on
  tdd : Outport
  wires:
  Gain/1 -> tdd/1
  Product/1 -> Gain/1
  E_diff_F/1 -> Product/3
  N_diff_F/1 -> Product/2
  T_g/1 -> Product/1

== system Pt_All_4WD_TS801/pt_model_4WD_ATMT/Front Differential /haibun/nejire ==
  W_err : Inport
  D_lock_F : Constant  Value=LOCKED_FD_DAMP
  Gain : Gain  Gain=-1  SaturateOnIntegerOverflow=on
  Integrator1 : Integrator
  K_lock_F : Constant  Value=LOCKED_FD_K
  Product : Product  SaturateOnIntegerOverflow=on  InputSameDT=on
  Product1 : Product  SaturateOnIntegerOverflow=on  InputSameDT=on
  Sum1 : Sum  Inputs=|++  SaturateOnIntegerOverflow=on  InputSameDT=on
  rad2deg : Gain  Gain=360/2/pi  SaturateOnIntegerOverflow=on
  T_lock_F : Outport
  wires:
  rad2deg/1 -> Integrator1/1, Product/1
  W_err/1 -> rad2deg/1
  Gain/1 -> T_lock_F/1
  Sum1/1 -> Gain/1
  D_lock_F/1 -> Product/2
  Integrator1/1 -> Product1/1
  K_lock_F/1 -> Product1/2
  Product1/1 -> Sum1/2
  Product/1 -> Sum1/1

== system Pt_All_4WD_TS801/pt_model_4WD_ATMT/Rear Differential/haibun/cal tdd ==
  N_diff_R : Inport
  T_g : Inport  Port=2
  E_diff_R : Inport  Port=3
  Gain : Gain  SaturateOnIntegerOverflow=on
  Product : Product  Inputs=3  SaturateOnIntegerOverflow=on  InputSameDT=on
  tdd : Outport
  wires:
  T_g/1 -> Product/1
  N_diff_R/1 -> Product/2
  E_diff_R/1 -> Product/3
  Product/1 -> Gain/1
  Gain/1 -> tdd/1

== system Pt_All_4WD_TS801/pt_model_4WD_ATMT/Rear Differential/haibun/nejire ==
  W_err : Inport
  D_lock_R : Constant  Value=LOCKED_RD_DAMP
  Gain : Gain  Gain=-1  SaturateOnIntegerOverflow=on
  Integrator1 : Integrator
  K_lock_R : Constant  Value=LOCKED_RD_K
  Product : Product  SaturateOnIntegerOverflow=on  InputSameDT=on
  Product1 : Product  SaturateOnIntegerOverflow=on  InputSameDT=on
  Sum1 : Sum  Inputs=|++  SaturateOnIntegerOverflow=on  InputSameDT=on
  rad2deg : Gain  Gain=360/2/pi  SaturateOnIntegerOverflow=on
  T_lock_R : Outport
  wires:
  rad2deg/1 -> Integrator1/1, Product/1
  W_err/1 -> rad2deg/1
  Product/1 -> Sum1/1
  Product1/1 -> Sum1/2
  K_lock_R/1 -> Product1/2
  Integrator1/1 -> Product1/1
  D_lock_R/1 -> Product/2
  Sum1/1 -> Gain/1
  Gain/1 -> T_lock_R/1
